simulink model "moduladorDelta"  (R2015a)
settings: Solver=ode45  StartTime=0.0  StopTime=1  MaxStep=0.02  RelTol=1e-3  AbsTol=0.02
settings Model: Creator=Javi  LastModifiedBy=Javi
settings SolverCC: InitialStep=0.02

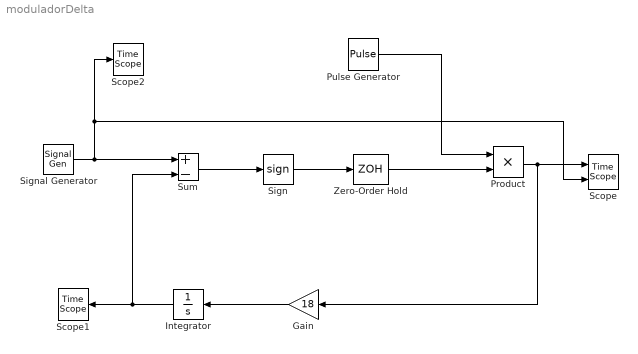
== system moduladorDelta ==
  Gain : Gain  Gain=18
  Integrator : Integrator  ZeroCross=off
  Product : Product
  Pulse Generator : DiscretePulseGenerator  PulseType=Time based  Period=0.02  PulseWidth=50
  Scope : TimeScope  NumInputPorts=2
  Scope1 : TimeScope
  Scope2 : TimeScope
  Sign : Signum  ZeroCross=off
  Signal Generator : SignalGenerator
  Sum : Sum  Inputs=+-
  Zero-Order Hold : ZeroOrderHold  SampleTime=0.02
  wires:
  Gain/1 -> Integrator/1
  Sum/1 -> Sign/1
  Sign/1 -> Zero-Order Hold/1
  Zero-Order Hold/1 -> Product/2
  Signal Generator/1 -> Sum/1, Scope/2, Scope2/1
  Integrator/1 -> Sum/2, Scope1/1
  Product/1 -> Gain/1, Scope/1
  Pulse Generator/1 -> Product/1
